simulink library "DTQC_lib"  (Simulink 7.5)
settings: Solver=ode45  StartTime=0.0  StopTime=10.0  RelTol=1e-3
values from neighbouring files (symbols this model uses):
  pDTQC_bool_AEBTrqSelect_C = Simulink.Parameter    [DTQC_par.m]
  pDTQC_Nm_ABSDelyOutTrq_C = Simulink.Parameter    [DTQC_par.m]
  pDTQC_Nm_AEBDelyOutTrq_C = Simulink.Parameter    [DTQC_par.m]
  pDTQC_Nm_AEBZeroTrq_C = Simulink.Parameter    [DTQC_par.m]
  pDTQC_Nm_ASRDelyOutTrq_C = Simulink.Parameter    [DTQC_par.m]
  pDTQC_Nm_MaxASRIntvTrq_C = Simulink.Parameter    [DTQC_par.m]
  pDTQC_Nm_MinASRIntvTrq_C = Simulink.Parameter    [DTQC_par.m]
  pDTQC_Nm_MSRDelyOutTrq_C = Simulink.Parameter    [DTQC_par.m]
  pDTQC_Nm_RBSDelyOutTrq_C = Simulink.Parameter    [DTQC_par.m]
  pDTQC_Nmps_ABSOutTrqLo_C = Simulink.Parameter    [DTQC_par.m]
  pDTQC_Nmps_ABSOutTrqUp_C = Simulink.Parameter    [DTQC_par.m]
  pDTQC_Nmps_AEBOutTrqLo_C = Simulink.Parameter    [DTQC_par.m]
  pDTQC_Nmps_AEBOutTrqUp_C = Simulink.Parameter    [DTQC_par.m]
  pDTQC_Nmps_ASROutTrqLo_C = Simulink.Parameter    [DTQC_par.m]
  pDTQC_Nmps_ASROutTrqUp_C = Simulink.Parameter    [DTQC_par.m]
  pDTQC_Nmps_MSROutTrqLo_C = Simulink.Parameter    [DTQC_par.m]
  pDTQC_Nmps_MSROutTrqUp_C = Simulink.Parameter    [DTQC_par.m]
  pDTQC_Nmps_RBSOutTrqLo_C = Simulink.Parameter    [DTQC_par.m]
  pDTQC_Nmps_RBSOutTrqUp_C = Simulink.Parameter    [DTQC_par.m]
libraries: BaseOperationLib_Browser x52, A0EV_Lib1 x9, simulink x1
settings Model: Creator=wuaibin  LastModifiedBy=wuaibin

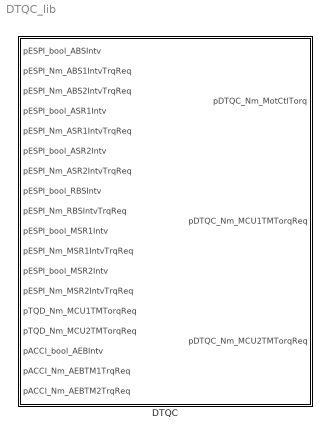
== system DTQC_lib ==
  DTQC : Subsystem  TreatAsAtomicUnit=on

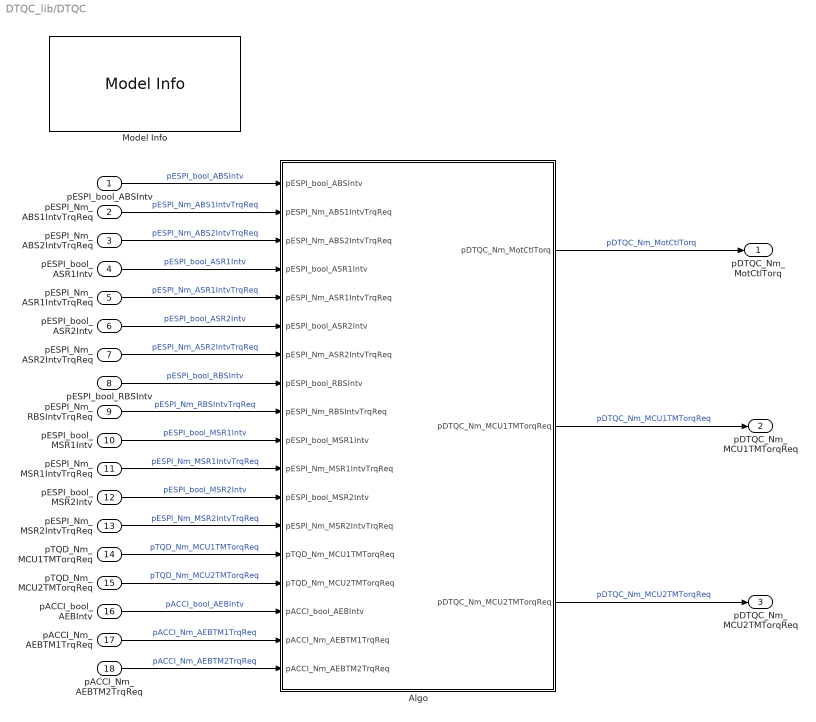
== system DTQC_lib/DTQC ==
  pESPI_bool_ABSIntv : Inport
  pESPI_Nm_ABS1IntvTrqReq : Inport  Port=2
  pESPI_Nm_ABS2IntvTrqReq : Inport  Port=3
  pESPI_bool_ASR1Intv : Inport  Port=4
  pESPI_Nm_ASR1IntvTrqReq : Inport  Port=5
  pESPI_bool_ASR2Intv : Inport  Port=6
  pESPI_Nm_ASR2IntvTrqReq : Inport  Port=7
  pESPI_bool_RBSIntv : Inport  Port=8
  pESPI_Nm_RBSIntvTrqReq : Inport  Port=9
  pESPI_bool_MSR1Intv : Inport  Port=10
  pESPI_Nm_MSR1IntvTrqReq : Inport  Port=11
  pESPI_bool_MSR2Intv : Inport  Port=12
  pESPI_Nm_MSR2IntvTrqReq : Inport  Port=13
  pTQD_Nm_MCU1TMTorqReq : Inport  Port=14
  pTQD_Nm_MCU2TMTorqReq : Inport  Port=15
  pACCI_bool_AEBIntv : Inport  Port=16
  pACCI_Nm_AEBTM1TrqReq : Inport  Port=17
  pACCI_Nm_AEBTM2TrqReq : Inport  Port=18
  Algo : Subsystem
  Model Info : simulink/Model-Wide Utilities/Model Info  SystemSampleTime=-1  InitialBlockCM=None  BlockCM=None  Frame=on  DisplayStringWithTags=Model Info\nCreated: %<Created>\nCreator: %<Creator>  HorizontalTextAlignment=Center  LeftAlignmentValue=0.5  SourceBlockDiagram=HQEV_HCU  TagMaxNumber=20
  pDTQC_Nm_MotCtlTorq : Outport  OutDataType=fixdt(1, 16)  OutScaling=2^0
  pDTQC_Nm_MCU1TMTorqReq : Outport  Port=2
  pDTQC_Nm_MCU2TMTorqReq : Outport  Port=3
  wires:
  pACCI_Nm_AEBTM2TrqReq/1 -> Algo/18(pACCI_Nm_AEBTM2TrqReq)  "pACCI_Nm_AEBTM2TrqReq"
  pACCI_Nm_AEBTM1TrqReq/1 -> Algo/17(pACCI_Nm_AEBTM1TrqReq)  "pACCI_Nm_AEBTM1TrqReq"
  pACCI_bool_AEBIntv/1 -> Algo/16(pACCI_bool_AEBIntv)  "pACCI_bool_AEBIntv"
  pTQD_Nm_MCU2TMTorqReq/1 -> Algo/15(pTQD_Nm_MCU2TMTorqReq)  "pTQD_Nm_MCU2TMTorqReq"
  pTQD_Nm_MCU1TMTorqReq/1 -> Algo/14(pTQD_Nm_MCU1TMTorqReq)  "pTQD_Nm_MCU1TMTorqReq"
  pESPI_Nm_MSR2IntvTrqReq/1 -> Algo/13(pESPI_Nm_MSR2IntvTrqReq)  "pESPI_Nm_MSR2IntvTrqReq"
  pESPI_bool_MSR2Intv/1 -> Algo/12(pESPI_bool_MSR2Intv)  "pESPI_bool_MSR2Intv"
  pESPI_Nm_MSR1IntvTrqReq/1 -> Algo/11(pESPI_Nm_MSR1IntvTrqReq)  "pESPI_Nm_MSR1IntvTrqReq"
  pESPI_bool_MSR1Intv/1 -> Algo/10(pESPI_bool_MSR1Intv)  "pESPI_bool_MSR1Intv"
  pESPI_Nm_RBSIntvTrqReq/1 -> Algo/9(pESPI_Nm_RBSIntvTrqReq)  "pESPI_Nm_RBSIntvTrqReq"
  pESPI_bool_RBSIntv/1 -> Algo/8(pESPI_bool_RBSIntv)  "pESPI_bool_RBSIntv"
  pESPI_Nm_ASR2IntvTrqReq/1 -> Algo/7(pESPI_Nm_ASR2IntvTrqReq)  "pESPI_Nm_ASR2IntvTrqReq"
  pESPI_bool_ASR2Intv/1 -> Algo/6(pESPI_bool_ASR2Intv)  "pESPI_bool_ASR2Intv"
  pESPI_Nm_ASR1IntvTrqReq/1 -> Algo/5(pESPI_Nm_ASR1IntvTrqReq)  "pESPI_Nm_ASR1IntvTrqReq"
  pESPI_bool_ASR1Intv/1 -> Algo/4(pESPI_bool_ASR1Intv)  "pESPI_bool_ASR1Intv"
  pESPI_Nm_ABS2IntvTrqReq/1 -> Algo/3(pESPI_Nm_ABS2IntvTrqReq)  "pESPI_Nm_ABS2IntvTrqReq"
  pESPI_Nm_ABS1IntvTrqReq/1 -> Algo/2(pESPI_Nm_ABS1IntvTrqReq)  "pESPI_Nm_ABS1IntvTrqReq"
  pESPI_bool_ABSIntv/1 -> Algo/1(pESPI_bool_ABSIntv)  "pESPI_bool_ABSIntv"
  Algo/3(pDTQC_Nm_MCU2TMTorqReq) -> pDTQC_Nm_MCU2TMTorqReq/1  "pDTQC_Nm_MCU2TMTorqReq"
  Algo/2(pDTQC_Nm_MCU1TMTorqReq) -> pDTQC_Nm_MCU1TMTorqReq/1  "pDTQC_Nm_MCU1TMTorqReq"
  Algo/1(pDTQC_Nm_MotCtlTorq) -> pDTQC_Nm_MotCtlTorq/1  "pDTQC_Nm_MotCtlTorq"

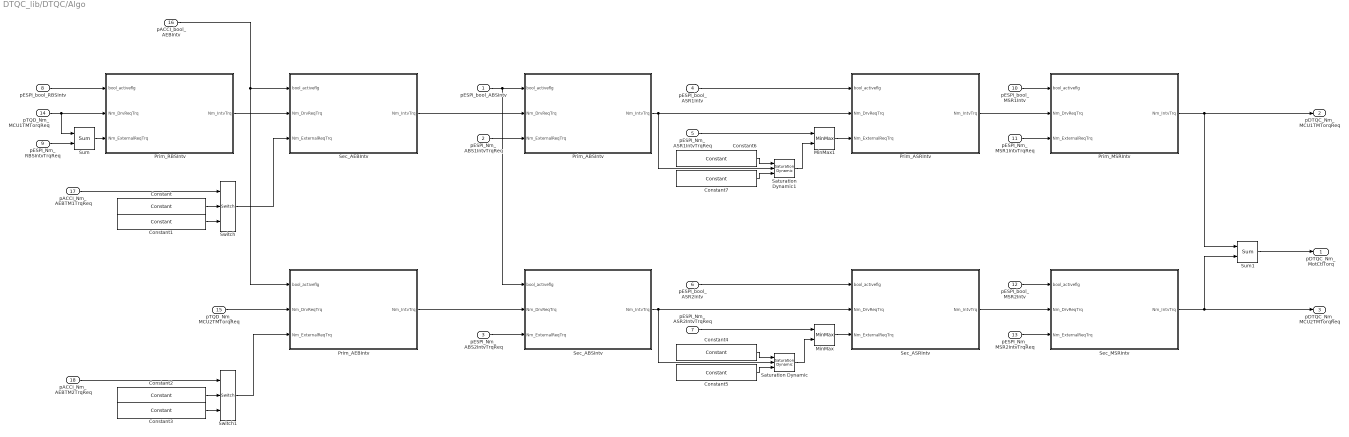
== system DTQC_lib/DTQC/Algo ==
  pESPI_bool_ABSIntv : Inport
  pESPI_Nm_ABS1IntvTrqReq : Inport  Port=2
  pESPI_Nm_ABS2IntvTrqReq : Inport  Port=3
  pESPI_bool_ASR1Intv : Inport  Port=4
  pESPI_Nm_ASR1IntvTrqReq : Inport  Port=5
  pESPI_bool_ASR2Intv : Inport  Port=6
  pESPI_Nm_ASR2IntvTrqReq : Inport  Port=7
  pESPI_bool_RBSIntv : Inport  Port=8
  pESPI_Nm_RBSIntvTrqReq : Inport  Port=9
  pESPI_bool_MSR1Intv : Inport  Port=10
  pESPI_Nm_MSR1IntvTrqReq : Inport  Port=11
  pESPI_bool_MSR2Intv : Inport  Port=12
  pESPI_Nm_MSR2IntvTrqReq : Inport  Port=13
  pTQD_Nm_MCU1TMTorqReq : Inport  Port=14
  pTQD_Nm_MCU2TMTorqReq : Inport  Port=15
  pACCI_bool_AEBIntv : Inport  Port=16
  pACCI_Nm_AEBTM1TrqReq : Inport  Port=17
  pACCI_Nm_AEBTM2TrqReq : Inport  Port=18
  Constant : BaseOperationLib_Browser/Sources&Sinks/Constant  Value=pDTQC_bool_AEBTrqSelect_C  OutMin=[]  OutMax=[]  OutDataType=fixdt(1, 16)  ConRadixGroup=Use specified scaling  OutScaling=2^0  OutDataTypeStr=Inherit: Inherit from 'Constant value'
  Constant1 : BaseOperationLib_Browser/Sources&Sinks/Constant  Value=pDTQC_Nm_AEBZeroTrq_C  OutMin=[]  OutMax=[]  OutDataType=fixdt(1, 16)  ConRadixGroup=Use specified scaling  OutScaling=2^0  OutDataTypeStr=Inherit: Inherit from 'Constant value'
  Constant2 : BaseOperationLib_Browser/Sources&Sinks/Constant  Value=pDTQC_bool_AEBTrqSelect_C  OutMin=[]  OutMax=[]  OutDataType=fixdt(1, 16)  ConRadixGroup=Use specified scaling  OutScaling=2^0  OutDataTypeStr=Inherit: Inherit from 'Constant value'
  Constant3 : BaseOperationLib_Browser/Sources&Sinks/Constant  Value=pDTQC_Nm_AEBZeroTrq_C  OutMin=[]  OutMax=[]  OutDataType=fixdt(1, 16)  ConRadixGroup=Use specified scaling  OutScaling=2^0  OutDataTypeStr=Inherit: Inherit from 'Constant value'
  Constant4 : BaseOperationLib_Browser/Sources&Sinks/Constant  Value=pDTQC_Nm_MaxASRIntvTrq_C  OutMin=[]  OutMax=[]  OutDataType=fixdt(1, 16)  ConRadixGroup=Use specified scaling  OutScaling=2^0  OutDataTypeStr=Inherit: Inherit from 'Constant value'
  Constant5 : BaseOperationLib_Browser/Sources&Sinks/Constant  Value=pDTQC_Nm_MinASRIntvTrq_C  OutMin=[]  OutMax=[]  OutDataType=fixdt(1, 16)  ConRadixGroup=Use specified scaling  OutScaling=2^0  OutDataTypeStr=Inherit: Inherit from 'Constant value'
  Constant6 : BaseOperationLib_Browser/Sources&Sinks/Constant  Value=pDTQC_Nm_MaxASRIntvTrq_C  OutMin=[]  OutMax=[]  OutDataType=fixdt(1, 16)  ConRadixGroup=Use specified scaling  OutScaling=2^0  OutDataTypeStr=Inherit: Inherit from 'Constant value'
  Constant7 : BaseOperationLib_Browser/Sources&Sinks/Constant  Value=pDTQC_Nm_MinASRIntvTrq_C  OutMin=[]  OutMax=[]  OutDataType=fixdt(1, 16)  ConRadixGroup=Use specified scaling  OutScaling=2^0  OutDataTypeStr=Inherit: Inherit from 'Constant value'
  MinMax : BaseOperationLib_Browser/Math Operations Changed/MinMax  Function=min  Inputs=2  InputSameDT=on  OutMin=[]  OutMax=[]  OutDataType=fixdt(1, 16)  OutScaling=2^0  SaturateOnIntegerOverflow=on
  MinMax1 : BaseOperationLib_Browser/Math Operations Changed/MinMax  Function=min  Inputs=2  InputSameDT=on  OutMin=[]  OutMax=[]  OutDataType=fixdt(1, 16)  OutScaling=2^0  SaturateOnIntegerOverflow=on
  Prim_ABSIntv : Subsystem
  Prim_AEBIntv : Subsystem
  Prim_ASRIntv : Subsystem
  Prim_MSRIntv : Subsystem
  Prim_RBSIntv : Subsystem
  Saturation Dynamic : BaseOperationLib_Browser/Discontinuities Unchanged/Saturation Dynamic  SystemSampleTime=-1  OutMin=[]  OutMax=[]  OutDataTypeStr=Inherit: Same as second input  OutDataType=fixdt(1, 16)  OutScaling=2^-10  DoSatur=on
  Saturation Dynamic1 : BaseOperationLib_Browser/Discontinuities Unchanged/Saturation Dynamic  SystemSampleTime=-1  OutMin=[]  OutMax=[]  OutDataTypeStr=Inherit: Same as second input  OutDataType=fixdt(1, 16)  OutScaling=2^-10  DoSatur=on
  Sec_ABSIntv : Subsystem
  Sec_AEBIntv : Subsystem
  Sec_ASRIntv : Subsystem
  Sec_MSRIntv : Subsystem
  Sum : BaseOperationLib_Browser/Math Operations Changed/Sum  Inputs=+-  InputSameDT=on  OutMin=[]  OutMax=[]  OutDataType=fixdt(1, 16)  OutScaling=2^0  SaturateOnIntegerOverflow=on
  Sum1 : BaseOperationLib_Browser/Math Operations Changed/Sum  Inputs=++  InputSameDT=on  OutMin=[]  OutMax=[]  OutDataType=fixdt(1, 16)  OutScaling=2^0  SaturateOnIntegerOverflow=on
  Switch : BaseOperationLib_Browser/Signal Routing Changed/Switch  Criteria=u2 ~= 0  Threshold=1  InputSameDT=on  OutMin=[]  OutMax=[]  OutDataType=fixdt(1,16,0)  OutScaling=[]  SaturateOnIntegerOverflow=on
  Switch1 : BaseOperationLib_Browser/Signal Routing Changed/Switch  Criteria=u2 ~= 0  Threshold=1  InputSameDT=on  OutMin=[]  OutMax=[]  OutDataType=fixdt(1,16,0)  OutScaling=[]  SaturateOnIntegerOverflow=on
  pDTQC_Nm_MotCtlTorq : Outport  OutDataType=fixdt(1, 16)  OutScaling=2^0
  pDTQC_Nm_MCU1TMTorqReq : Outport  Port=2
  pDTQC_Nm_MCU2TMTorqReq : Outport  Port=3
  wires:
  pESPI_Nm_ASR1IntvTrqReq/1 -> MinMax1/1
  Saturation Dynamic1/1 -> MinMax1/2
  Constant7/1 -> Saturation Dynamic1/3
  Constant6/1 -> Saturation Dynamic1/1
  MinMax1/1 -> Prim_ASRIntv/3(Nm_ExternalReqTrq)
  Constant5/1 -> Saturation Dynamic/3
  Constant4/1 -> Saturation Dynamic/1
  MinMax/1 -> Sec_ASRIntv/3(Nm_ExternalReqTrq)
  Saturation Dynamic/1 -> MinMax/2
  pESPI_Nm_ASR2IntvTrqReq/1 -> MinMax/1
  Sec_ASRIntv/1(Nm_IntvTrq) -> Sec_MSRIntv/2(Nm_DrvReqTrq)
  pESPI_bool_ASR2Intv/1 -> Sec_ASRIntv/1(bool_activeflg)
  pESPI_Nm_ABS2IntvTrqReq/1 -> Sec_ABSIntv/3(Nm_ExternalReqTrq)
  Prim_AEBIntv/1(Nm_IntvTrq) -> Sec_ABSIntv/2(Nm_DrvReqTrq)
  Sec_ABSIntv/1(Nm_IntvTrq) -> Saturation Dynamic/2, Sec_ASRIntv/2(Nm_DrvReqTrq)
  Prim_ASRIntv/1(Nm_IntvTrq) -> Prim_MSRIntv/2(Nm_DrvReqTrq)
  pESPI_bool_ASR1Intv/1 -> Prim_ASRIntv/1(bool_activeflg)
  Sec_AEBIntv/1(Nm_IntvTrq) -> Prim_ABSIntv/2(Nm_DrvReqTrq)
  Prim_ABSIntv/1(Nm_IntvTrq) -> Saturation Dynamic1/2, Prim_ASRIntv/2(Nm_DrvReqTrq)
  pESPI_Nm_ABS1IntvTrqReq/1 -> Prim_ABSIntv/3(Nm_ExternalReqTrq)
  pESPI_bool_ABSIntv/1 -> Sec_ABSIntv/1(bool_activeflg), Prim_ABSIntv/1(bool_activeflg)
  Sec_MSRIntv/1(Nm_IntvTrq) -> pDTQC_Nm_MCU2TMTorqReq/1, Sum1/2
  Prim_MSRIntv/1(Nm_IntvTrq) -> Sum1/1, pDTQC_Nm_MCU1TMTorqReq/1
  Switch1/1 -> Prim_AEBIntv/3(Nm_ExternalReqTrq)
  Switch/1 -> Sec_AEBIntv/3(Nm_ExternalReqTrq)
  pACCI_bool_AEBIntv/1 -> Prim_AEBIntv/1(bool_activeflg), Sec_AEBIntv/1(bool_activeflg)
  pTQD_Nm_MCU2TMTorqReq/1 -> Prim_AEBIntv/2(Nm_DrvReqTrq)
  Prim_RBSIntv/1(Nm_IntvTrq) -> Sec_AEBIntv/2(Nm_DrvReqTrq)
  Sum1/1 -> pDTQC_Nm_MotCtlTorq/1
  pESPI_Nm_MSR2IntvTrqReq/1 -> Sec_MSRIntv/3(Nm_ExternalReqTrq)
  pESPI_bool_MSR2Intv/1 -> Sec_MSRIntv/1(bool_activeflg)
  Constant3/1 -> Switch1/3
  pACCI_Nm_AEBTM2TrqReq/1 -> Switch1/1
  Constant2/1 -> Switch1/2
  Constant1/1 -> Switch/3
  pACCI_Nm_AEBTM1TrqReq/1 -> Switch/1
  Constant/1 -> Switch/2
  pESPI_Nm_RBSIntvTrqReq/1 -> Sum/2
  Sum/1 -> Prim_RBSIntv/3(Nm_ExternalReqTrq)
  pESPI_Nm_MSR1IntvTrqReq/1 -> Prim_MSRIntv/3(Nm_ExternalReqTrq)
  pESPI_bool_MSR1Intv/1 -> Prim_MSRIntv/1(bool_activeflg)
  pESPI_bool_RBSIntv/1 -> Prim_RBSIntv/1(bool_activeflg)
  pTQD_Nm_MCU1TMTorqReq/1 -> Sum/1, Prim_RBSIntv/2(Nm_DrvReqTrq)

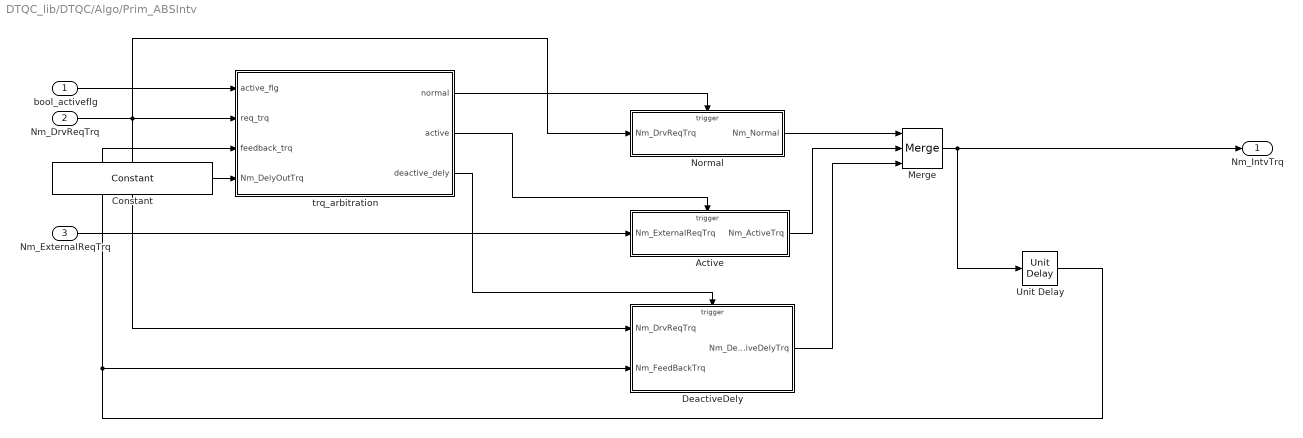
== system DTQC_lib/DTQC/Algo/Prim_ABSIntv ==
  bool_activeflg : Inport
  Nm_DrvReqTrq : Inport  Port=2
  Nm_ExternalReqTrq : Inport  Port=3
  Active : Subsystem
  Constant : BaseOperationLib_Browser/Sources&Sinks/Constant  Value=pDTQC_Nm_ABSDelyOutTrq_C  OutMin=[]  OutMax=[]  OutDataType=fixdt(1, 16)  ConRadixGroup=Use specified scaling  OutScaling=2^0  OutDataTypeStr=Inherit: Inherit from 'Constant value'
  DeactiveDely : Subsystem
  Merge : Merge  Inputs=3
  Normal : Subsystem
  Unit Delay : BaseOperationLib_Browser/Discrete Unchanged /Unit Delay  X0=0  SampleTime=-1
  trq_arbitration : Stateflow chart  TreatAsAtomicUnit=on
  Nm_IntvTrq : Outport  OutDataType=fixdt(1, 16)  OutScaling=2^0
  wires:
  bool_activeflg/1 -> trq_arbitration/1(active_flg)
  Nm_DrvReqTrq/1 -> trq_arbitration/2(req_trq), Normal/1(Nm_DrvReqTrq), DeactiveDely/1(Nm_DrvReqTrq)
  trq_arbitration/1(normal) -> Normal/Trigger
  trq_arbitration/2(active) -> Active/Trigger
  trq_arbitration/3(deactive_dely) -> DeactiveDely/Trigger
  Normal/1(Nm_Normal) -> Merge/1
  Active/1(Nm_ActiveTrq) -> Merge/2
  DeactiveDely/1(Nm_DeactiveDelyTrq) -> Merge/3
  Merge/1 -> Unit Delay/1, Nm_IntvTrq/1
  Unit Delay/1 -> trq_arbitration/3(feedback_trq), DeactiveDely/2(Nm_FeedBackTrq)
  Nm_ExternalReqTrq/1 -> Active/1(Nm_ExternalReqTrq)
  Constant/1 -> trq_arbitration/4(Nm_DelyOutTrq)

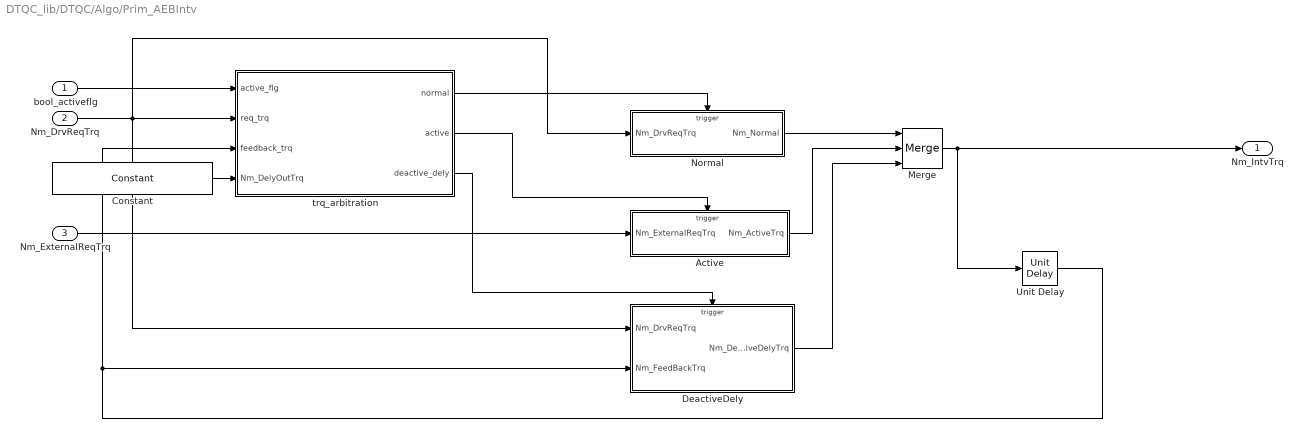
== system DTQC_lib/DTQC/Algo/Prim_AEBIntv ==
  bool_activeflg : Inport
  Nm_DrvReqTrq : Inport  Port=2
  Nm_ExternalReqTrq : Inport  Port=3
  Active : Subsystem
  Constant : BaseOperationLib_Browser/Sources&Sinks/Constant  Value=pDTQC_Nm_AEBDelyOutTrq_C  OutMin=[]  OutMax=[]  OutDataType=fixdt(1, 16)  ConRadixGroup=Use specified scaling  OutScaling=2^0  OutDataTypeStr=Inherit: Inherit from 'Constant value'
  DeactiveDely : Subsystem
  Merge : Merge  Inputs=3
  Normal : Subsystem
  Unit Delay : BaseOperationLib_Browser/Discrete Unchanged /Unit Delay  X0=0  SampleTime=-1
  trq_arbitration : Stateflow chart  TreatAsAtomicUnit=on
  Nm_IntvTrq : Outport  OutDataType=fixdt(1, 16)  OutScaling=2^0
  wires:
  Constant/1 -> trq_arbitration/4(Nm_DelyOutTrq)
  Nm_ExternalReqTrq/1 -> Active/1(Nm_ExternalReqTrq)
  Unit Delay/1 -> DeactiveDely/2(Nm_FeedBackTrq), trq_arbitration/3(feedback_trq)
  Merge/1 -> Nm_IntvTrq/1, Unit Delay/1
  DeactiveDely/1(Nm_DeactiveDelyTrq) -> Merge/3
  Active/1(Nm_ActiveTrq) -> Merge/2
  Normal/1(Nm_Normal) -> Merge/1
  trq_arbitration/3(deactive_dely) -> DeactiveDely/Trigger
  trq_arbitration/2(active) -> Active/Trigger
  trq_arbitration/1(normal) -> Normal/Trigger
  Nm_DrvReqTrq/1 -> DeactiveDely/1(Nm_DrvReqTrq), Normal/1(Nm_DrvReqTrq), trq_arbitration/2(req_trq)
  bool_activeflg/1 -> trq_arbitration/1(active_flg)

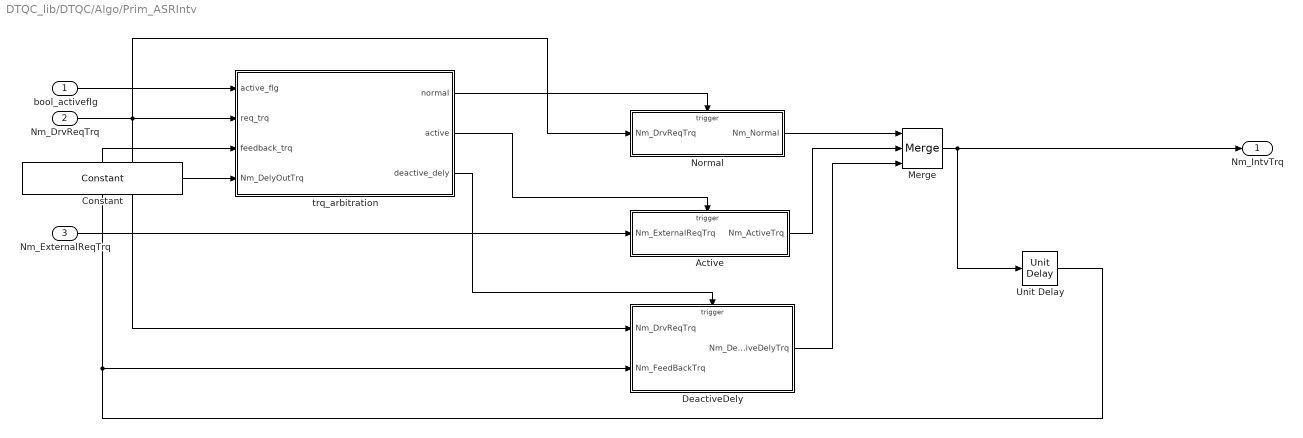
== system DTQC_lib/DTQC/Algo/Prim_ASRIntv ==
  bool_activeflg : Inport
  Nm_DrvReqTrq : Inport  Port=2
  Nm_ExternalReqTrq : Inport  Port=3
  Active : Subsystem
  Constant : BaseOperationLib_Browser/Sources&Sinks/Constant  Value=pDTQC_Nm_ASRDelyOutTrq_C  OutMin=[]  OutMax=[]  OutDataType=fixdt(1, 16)  ConRadixGroup=Use specified scaling  OutScaling=2^0  OutDataTypeStr=Inherit: Inherit from 'Constant value'
  DeactiveDely : Subsystem
  Merge : Merge  Inputs=3
  Normal : Subsystem
  Unit Delay : BaseOperationLib_Browser/Discrete Unchanged /Unit Delay  X0=0  SampleTime=-1
  trq_arbitration : Stateflow chart  TreatAsAtomicUnit=on
  Nm_IntvTrq : Outport  OutDataType=fixdt(1, 16)  OutScaling=2^0
  wires:
  Constant/1 -> trq_arbitration/4(Nm_DelyOutTrq)
  Nm_ExternalReqTrq/1 -> Active/1(Nm_ExternalReqTrq)
  Unit Delay/1 -> DeactiveDely/2(Nm_FeedBackTrq), trq_arbitration/3(feedback_trq)
  Merge/1 -> Nm_IntvTrq/1, Unit Delay/1
  DeactiveDely/1(Nm_DeactiveDelyTrq) -> Merge/3
  Active/1(Nm_ActiveTrq) -> Merge/2
  Normal/1(Nm_Normal) -> Merge/1
  trq_arbitration/3(deactive_dely) -> DeactiveDely/Trigger
  trq_arbitration/2(active) -> Active/Trigger
  trq_arbitration/1(normal) -> Normal/Trigger
  Nm_DrvReqTrq/1 -> DeactiveDely/1(Nm_DrvReqTrq), Normal/1(Nm_DrvReqTrq), trq_arbitration/2(req_trq)
  bool_activeflg/1 -> trq_arbitration/1(active_flg)

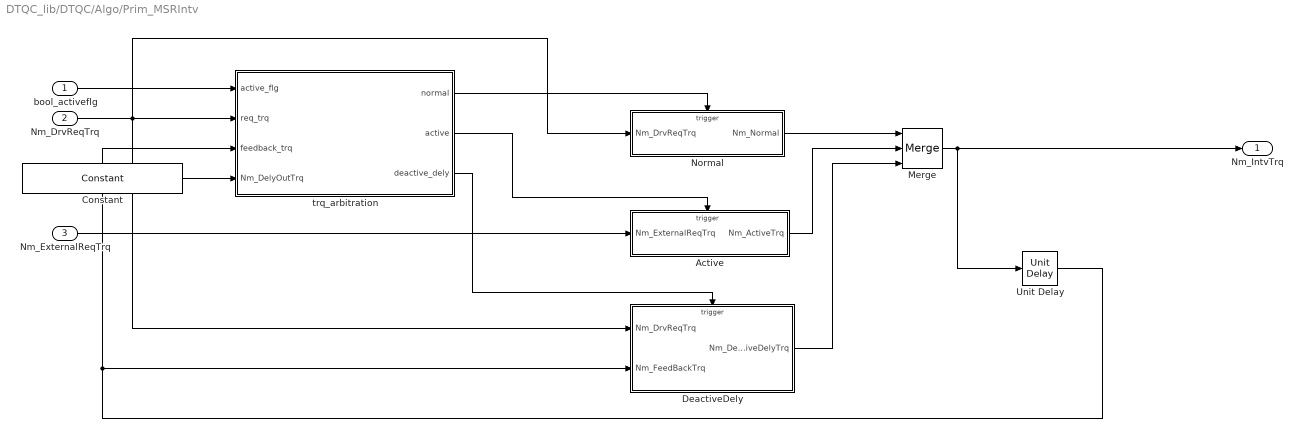
== system DTQC_lib/DTQC/Algo/Prim_MSRIntv ==
  bool_activeflg : Inport
  Nm_DrvReqTrq : Inport  Port=2
  Nm_ExternalReqTrq : Inport  Port=3
  Active : Subsystem
  Constant : BaseOperationLib_Browser/Sources&Sinks/Constant  Value=pDTQC_Nm_MSRDelyOutTrq_C  OutMin=[]  OutMax=[]  OutDataType=fixdt(1, 16)  ConRadixGroup=Use specified scaling  OutScaling=2^0  OutDataTypeStr=Inherit: Inherit from 'Constant value'
  DeactiveDely : Subsystem
  Merge : Merge  Inputs=3
  Normal : Subsystem
  Unit Delay : BaseOperationLib_Browser/Discrete Unchanged /Unit Delay  X0=0  SampleTime=-1
  trq_arbitration : Stateflow chart  TreatAsAtomicUnit=on
  Nm_IntvTrq : Outport  OutDataType=fixdt(1, 16)  OutScaling=2^0
  wires:
  bool_activeflg/1 -> trq_arbitration/1(active_flg)
  Nm_DrvReqTrq/1 -> trq_arbitration/2(req_trq), Normal/1(Nm_DrvReqTrq), DeactiveDely/1(Nm_DrvReqTrq)
  trq_arbitration/1(normal) -> Normal/Trigger
  trq_arbitration/2(active) -> Active/Trigger
  trq_arbitration/3(deactive_dely) -> DeactiveDely/Trigger
  Normal/1(Nm_Normal) -> Merge/1
  Active/1(Nm_ActiveTrq) -> Merge/2
  DeactiveDely/1(Nm_DeactiveDelyTrq) -> Merge/3
  Merge/1 -> Unit Delay/1, Nm_IntvTrq/1
  Unit Delay/1 -> trq_arbitration/3(feedback_trq), DeactiveDely/2(Nm_FeedBackTrq)
  Nm_ExternalReqTrq/1 -> Active/1(Nm_ExternalReqTrq)
  Constant/1 -> trq_arbitration/4(Nm_DelyOutTrq)

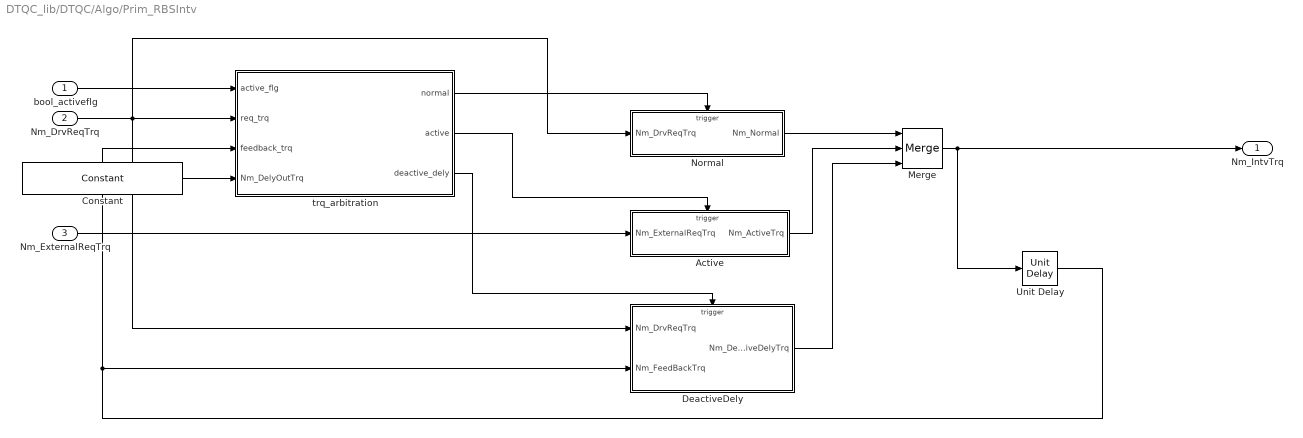
== system DTQC_lib/DTQC/Algo/Prim_RBSIntv ==
  bool_activeflg : Inport
  Nm_DrvReqTrq : Inport  Port=2
  Nm_ExternalReqTrq : Inport  Port=3
  Active : Subsystem
  Constant : BaseOperationLib_Browser/Sources&Sinks/Constant  Value=pDTQC_Nm_RBSDelyOutTrq_C  OutMin=[]  OutMax=[]  OutDataType=fixdt(1, 16)  ConRadixGroup=Use specified scaling  OutScaling=2^0  OutDataTypeStr=Inherit: Inherit from 'Constant value'
  DeactiveDely : Subsystem
  Merge : Merge  Inputs=3
  Normal : Subsystem
  Unit Delay : BaseOperationLib_Browser/Discrete Unchanged /Unit Delay  X0=0  SampleTime=-1
  trq_arbitration : Stateflow chart  TreatAsAtomicUnit=on
  Nm_IntvTrq : Outport  OutDataType=fixdt(1, 16)  OutScaling=2^0
  wires:
  Constant/1 -> trq_arbitration/4(Nm_DelyOutTrq)
  Nm_ExternalReqTrq/1 -> Active/1(Nm_ExternalReqTrq)
  Unit Delay/1 -> DeactiveDely/2(Nm_FeedBackTrq), trq_arbitration/3(feedback_trq)
  Merge/1 -> Nm_IntvTrq/1, Unit Delay/1
  DeactiveDely/1(Nm_DeactiveDelyTrq) -> Merge/3
  Active/1(Nm_ActiveTrq) -> Merge/2
  Normal/1(Nm_Normal) -> Merge/1
  trq_arbitration/3(deactive_dely) -> DeactiveDely/Trigger
  trq_arbitration/2(active) -> Active/Trigger
  trq_arbitration/1(normal) -> Normal/Trigger
  Nm_DrvReqTrq/1 -> DeactiveDely/1(Nm_DrvReqTrq), Normal/1(Nm_DrvReqTrq), trq_arbitration/2(req_trq)
  bool_activeflg/1 -> trq_arbitration/1(active_flg)

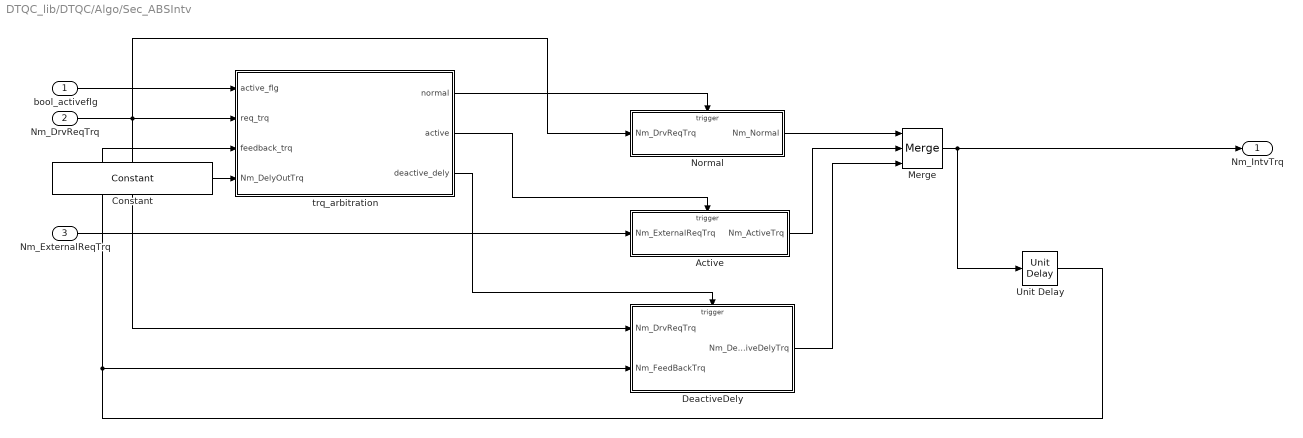
== system DTQC_lib/DTQC/Algo/Sec_ABSIntv ==
  bool_activeflg : Inport
  Nm_DrvReqTrq : Inport  Port=2
  Nm_ExternalReqTrq : Inport  Port=3
  Active : Subsystem
  Constant : BaseOperationLib_Browser/Sources&Sinks/Constant  Value=pDTQC_Nm_ABSDelyOutTrq_C  OutMin=[]  OutMax=[]  OutDataType=fixdt(1, 16)  ConRadixGroup=Use specified scaling  OutScaling=2^0  OutDataTypeStr=Inherit: Inherit from 'Constant value'
  DeactiveDely : Subsystem
  Merge : Merge  Inputs=3
  Normal : Subsystem
  Unit Delay : BaseOperationLib_Browser/Discrete Unchanged /Unit Delay  X0=0  SampleTime=-1
  trq_arbitration : Stateflow chart  TreatAsAtomicUnit=on
  Nm_IntvTrq : Outport  OutDataType=fixdt(1, 16)  OutScaling=2^0
  wires:
  Constant/1 -> trq_arbitration/4(Nm_DelyOutTrq)
  Nm_ExternalReqTrq/1 -> Active/1(Nm_ExternalReqTrq)
  Unit Delay/1 -> DeactiveDely/2(Nm_FeedBackTrq), trq_arbitration/3(feedback_trq)
  Merge/1 -> Nm_IntvTrq/1, Unit Delay/1
  DeactiveDely/1(Nm_DeactiveDelyTrq) -> Merge/3
  Active/1(Nm_ActiveTrq) -> Merge/2
  Normal/1(Nm_Normal) -> Merge/1
  trq_arbitration/3(deactive_dely) -> DeactiveDely/Trigger
  trq_arbitration/2(active) -> Active/Trigger
  trq_arbitration/1(normal) -> Normal/Trigger
  Nm_DrvReqTrq/1 -> DeactiveDely/1(Nm_DrvReqTrq), Normal/1(Nm_DrvReqTrq), trq_arbitration/2(req_trq)
  bool_activeflg/1 -> trq_arbitration/1(active_flg)

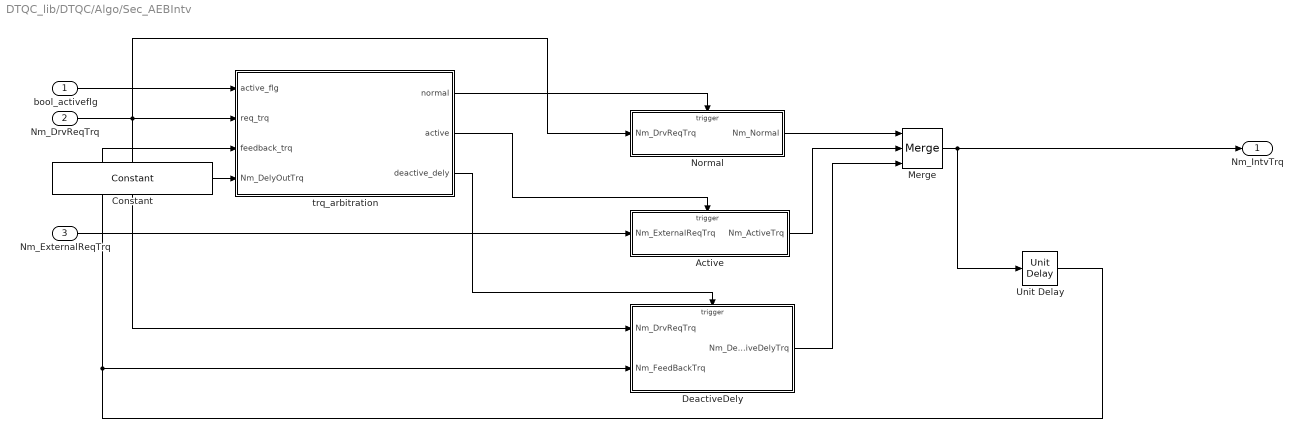
== system DTQC_lib/DTQC/Algo/Sec_AEBIntv ==
  bool_activeflg : Inport
  Nm_DrvReqTrq : Inport  Port=2
  Nm_ExternalReqTrq : Inport  Port=3
  Active : Subsystem
  Constant : BaseOperationLib_Browser/Sources&Sinks/Constant  Value=pDTQC_Nm_AEBDelyOutTrq_C  OutMin=[]  OutMax=[]  OutDataType=fixdt(1, 16)  ConRadixGroup=Use specified scaling  OutScaling=2^0  OutDataTypeStr=Inherit: Inherit from 'Constant value'
  DeactiveDely : Subsystem
  Merge : Merge  Inputs=3
  Normal : Subsystem
  Unit Delay : BaseOperationLib_Browser/Discrete Unchanged /Unit Delay  X0=0  SampleTime=-1
  trq_arbitration : Stateflow chart  TreatAsAtomicUnit=on
  Nm_IntvTrq : Outport  OutDataType=fixdt(1, 16)  OutScaling=2^0
  wires:
  bool_activeflg/1 -> trq_arbitration/1(active_flg)
  Nm_DrvReqTrq/1 -> trq_arbitration/2(req_trq), Normal/1(Nm_DrvReqTrq), DeactiveDely/1(Nm_DrvReqTrq)
  trq_arbitration/1(normal) -> Normal/Trigger
  trq_arbitration/2(active) -> Active/Trigger
  trq_arbitration/3(deactive_dely) -> DeactiveDely/Trigger
  Normal/1(Nm_Normal) -> Merge/1
  Active/1(Nm_ActiveTrq) -> Merge/2
  DeactiveDely/1(Nm_DeactiveDelyTrq) -> Merge/3
  Merge/1 -> Unit Delay/1, Nm_IntvTrq/1
  Unit Delay/1 -> trq_arbitration/3(feedback_trq), DeactiveDely/2(Nm_FeedBackTrq)
  Nm_ExternalReqTrq/1 -> Active/1(Nm_ExternalReqTrq)
  Constant/1 -> trq_arbitration/4(Nm_DelyOutTrq)

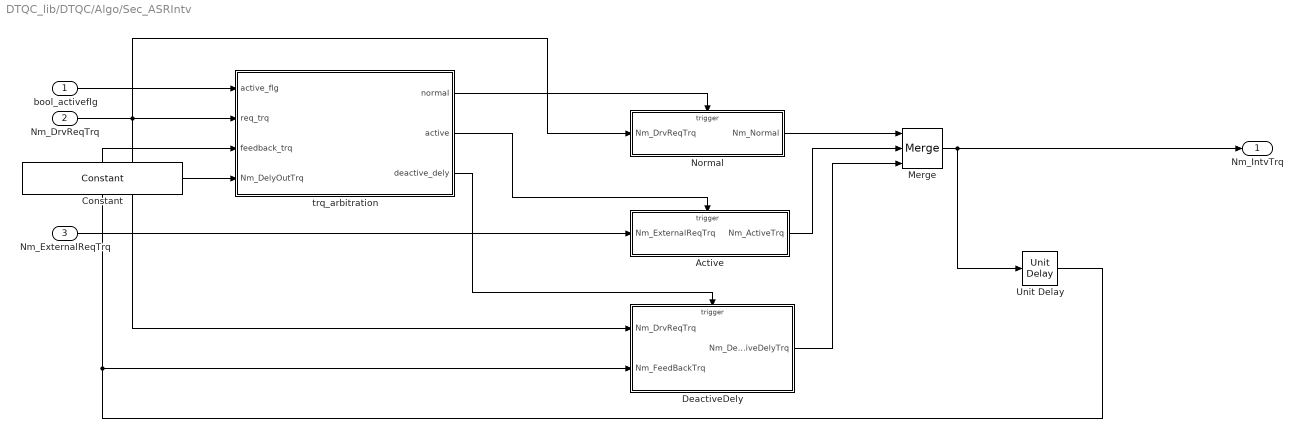
== system DTQC_lib/DTQC/Algo/Sec_ASRIntv ==
  bool_activeflg : Inport
  Nm_DrvReqTrq : Inport  Port=2
  Nm_ExternalReqTrq : Inport  Port=3
  Active : Subsystem
  Constant : BaseOperationLib_Browser/Sources&Sinks/Constant  Value=pDTQC_Nm_ASRDelyOutTrq_C  OutMin=[]  OutMax=[]  OutDataType=fixdt(1, 16)  ConRadixGroup=Use specified scaling  OutScaling=2^0  OutDataTypeStr=Inherit: Inherit from 'Constant value'
  DeactiveDely : Subsystem
  Merge : Merge  Inputs=3
  Normal : Subsystem
  Unit Delay : BaseOperationLib_Browser/Discrete Unchanged /Unit Delay  X0=0  SampleTime=-1
  trq_arbitration : Stateflow chart  TreatAsAtomicUnit=on
  Nm_IntvTrq : Outport  OutDataType=fixdt(1, 16)  OutScaling=2^0
  wires:
  bool_activeflg/1 -> trq_arbitration/1(active_flg)
  Nm_DrvReqTrq/1 -> trq_arbitration/2(req_trq), Normal/1(Nm_DrvReqTrq), DeactiveDely/1(Nm_DrvReqTrq)
  trq_arbitration/1(normal) -> Normal/Trigger
  trq_arbitration/2(active) -> Active/Trigger
  trq_arbitration/3(deactive_dely) -> DeactiveDely/Trigger
  Normal/1(Nm_Normal) -> Merge/1
  Active/1(Nm_ActiveTrq) -> Merge/2
  DeactiveDely/1(Nm_DeactiveDelyTrq) -> Merge/3
  Merge/1 -> Unit Delay/1, Nm_IntvTrq/1
  Unit Delay/1 -> trq_arbitration/3(feedback_trq), DeactiveDely/2(Nm_FeedBackTrq)
  Nm_ExternalReqTrq/1 -> Active/1(Nm_ExternalReqTrq)
  Constant/1 -> trq_arbitration/4(Nm_DelyOutTrq)

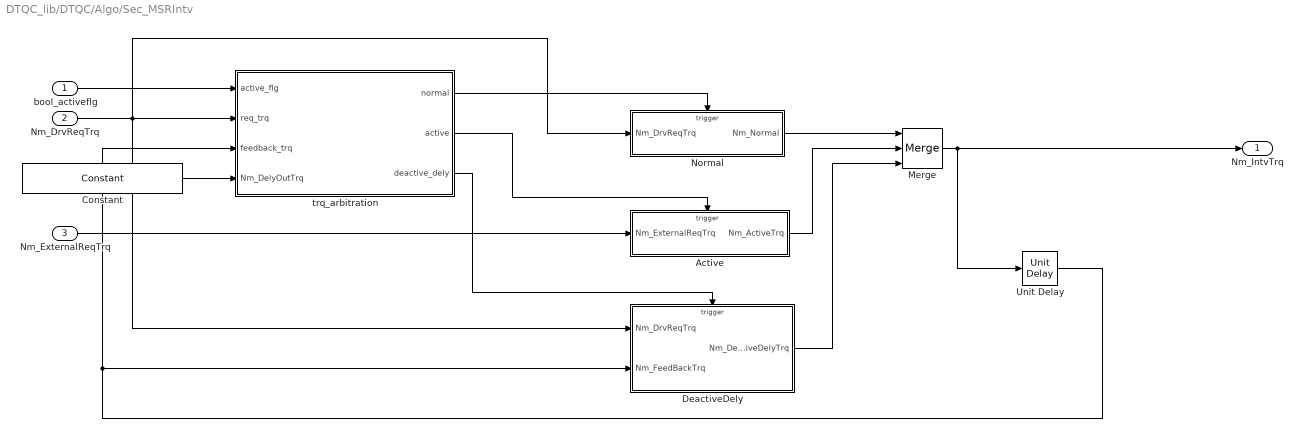
== system DTQC_lib/DTQC/Algo/Sec_MSRIntv ==
  bool_activeflg : Inport
  Nm_DrvReqTrq : Inport  Port=2
  Nm_ExternalReqTrq : Inport  Port=3
  Active : Subsystem
  Constant : BaseOperationLib_Browser/Sources&Sinks/Constant  Value=pDTQC_Nm_MSRDelyOutTrq_C  OutMin=[]  OutMax=[]  OutDataType=fixdt(1, 16)  ConRadixGroup=Use specified scaling  OutScaling=2^0  OutDataTypeStr=Inherit: Inherit from 'Constant value'
  DeactiveDely : Subsystem
  Merge : Merge  Inputs=3
  Normal : Subsystem
  Unit Delay : BaseOperationLib_Browser/Discrete Unchanged /Unit Delay  X0=0  SampleTime=-1
  trq_arbitration : Stateflow chart  TreatAsAtomicUnit=on
  Nm_IntvTrq : Outport  OutDataType=fixdt(1, 16)  OutScaling=2^0
  wires:
  Constant/1 -> trq_arbitration/4(Nm_DelyOutTrq)
  Nm_ExternalReqTrq/1 -> Active/1(Nm_ExternalReqTrq)
  Unit Delay/1 -> DeactiveDely/2(Nm_FeedBackTrq), trq_arbitration/3(feedback_trq)
  Merge/1 -> Nm_IntvTrq/1, Unit Delay/1
  DeactiveDely/1(Nm_DeactiveDelyTrq) -> Merge/3
  Active/1(Nm_ActiveTrq) -> Merge/2
  Normal/1(Nm_Normal) -> Merge/1
  trq_arbitration/3(deactive_dely) -> DeactiveDely/Trigger
  trq_arbitration/2(active) -> Active/Trigger
  trq_arbitration/1(normal) -> Normal/Trigger
  Nm_DrvReqTrq/1 -> DeactiveDely/1(Nm_DrvReqTrq), Normal/1(Nm_DrvReqTrq), trq_arbitration/2(req_trq)
  bool_activeflg/1 -> trq_arbitration/1(active_flg)

== system DTQC_lib/DTQC/Algo/Prim_ABSIntv/Active ==
  Nm_ExternalReqTrq : Inport  OutDataType=fixdt(1, 16)  OutScaling=2^0
  function : TriggerPort  TriggerType=function-call
  Nm_ActiveTrq : Outport  OutDataType=fixdt(1, 16)  OutScaling=2^0
  wires:
  Nm_ExternalReqTrq/1 -> Nm_ActiveTrq/1

== system DTQC_lib/DTQC/Algo/Prim_ABSIntv/DeactiveDely ==
  Nm_DrvReqTrq : Inport  OutDataType=fixdt(1, 16)  OutScaling=2^0
  Nm_FeedBackTrq : Inport  Port=2  OutDataType=fixdt(1, 16)  OutScaling=2^0
  function : TriggerPort  TriggerType=function-call
  Constant : BaseOperationLib_Browser/Sources&Sinks/Constant  Value=pDTQC_Nmps_ABSOutTrqUp_C  OutMin=[]  OutMax=[]  OutDataType=fixdt(1, 16)  ConRadixGroup=Use specified scaling  OutScaling=2^0  OutDataTypeStr=Inherit: Inherit from 'Constant value'
  Constant1 : BaseOperationLib_Browser/Sources&Sinks/Constant  Value=pDTQC_Nmps_ABSOutTrqLo_C  OutMin=[]  OutMax=[]  OutDataType=fixdt(1, 16)  ConRadixGroup=Use specified scaling  OutScaling=2^0  OutDataTypeStr=Inherit: Inherit from 'Constant value'
  RampLim : A0EV_Lib1/Filter & Ramp/RampLim  SystemSampleTime=-1
  Nm_DeactiveDelyTrq : Outport  OutDataType=fixdt(1, 16)  OutScaling=2^0
  wires:
  Nm_DrvReqTrq/1 -> RampLim/1
  Nm_FeedBackTrq/1 -> RampLim/2
  RampLim/1 -> Nm_DeactiveDelyTrq/1
  Constant/1 -> RampLim/3
  Constant1/1 -> RampLim/4

== system DTQC_lib/DTQC/Algo/Prim_ABSIntv/Normal ==
  Nm_DrvReqTrq : Inport  OutDataType=fixdt(1, 16)  OutScaling=2^0
  function : TriggerPort  TriggerType=function-call
  Nm_Normal : Outport  OutDataType=fixdt(1, 16)  OutScaling=2^0
  wires:
  Nm_DrvReqTrq/1 -> Nm_Normal/1

== system DTQC_lib/DTQC/Algo/Prim_AEBIntv/Active ==
  Nm_ExternalReqTrq : Inport  OutDataType=fixdt(1, 16)  OutScaling=2^0
  function : TriggerPort  TriggerType=function-call
  Nm_ActiveTrq : Outport  OutDataType=fixdt(1, 16)  OutScaling=2^0
  wires:
  Nm_ExternalReqTrq/1 -> Nm_ActiveTrq/1

== system DTQC_lib/DTQC/Algo/Prim_AEBIntv/DeactiveDely ==
  Nm_DrvReqTrq : Inport  OutDataType=fixdt(1, 16)  OutScaling=2^0
  Nm_FeedBackTrq : Inport  Port=2  OutDataType=fixdt(1, 16)  OutScaling=2^0
  function : TriggerPort  TriggerType=function-call
  Constant : BaseOperationLib_Browser/Sources&Sinks/Constant  Value=pDTQC_Nmps_AEBOutTrqUp_C  OutMin=[]  OutMax=[]  OutDataType=fixdt(1, 16)  ConRadixGroup=Use specified scaling  OutScaling=2^0  OutDataTypeStr=Inherit: Inherit from 'Constant value'
  Constant1 : BaseOperationLib_Browser/Sources&Sinks/Constant  Value=pDTQC_Nmps_AEBOutTrqLo_C  OutMin=[]  OutMax=[]  OutDataType=fixdt(1, 16)  ConRadixGroup=Use specified scaling  OutScaling=2^0  OutDataTypeStr=Inherit: Inherit from 'Constant value'
  RampLim : A0EV_Lib1/Filter & Ramp/RampLim  SystemSampleTime=-1
  Nm_DeactiveDelyTrq : Outport  OutDataType=fixdt(1, 16)  OutScaling=2^0
  wires:
  Constant1/1 -> RampLim/4
  Constant/1 -> RampLim/3
  RampLim/1 -> Nm_DeactiveDelyTrq/1
  Nm_FeedBackTrq/1 -> RampLim/2
  Nm_DrvReqTrq/1 -> RampLim/1

== system DTQC_lib/DTQC/Algo/Prim_AEBIntv/Normal ==
  Nm_DrvReqTrq : Inport  OutDataType=fixdt(1, 16)  OutScaling=2^0
  function : TriggerPort  TriggerType=function-call
  Nm_Normal : Outport  OutDataType=fixdt(1, 16)  OutScaling=2^0
  wires:
  Nm_DrvReqTrq/1 -> Nm_Normal/1

== system DTQC_lib/DTQC/Algo/Prim_ASRIntv/Active ==
  Nm_ExternalReqTrq : Inport  OutDataType=fixdt(1, 16)  OutScaling=2^0
  function : TriggerPort  TriggerType=function-call
  Nm_ActiveTrq : Outport  OutDataType=fixdt(1, 16)  OutScaling=2^0
  wires:
  Nm_ExternalReqTrq/1 -> Nm_ActiveTrq/1

== system DTQC_lib/DTQC/Algo/Prim_ASRIntv/DeactiveDely ==
  Nm_DrvReqTrq : Inport  OutDataType=fixdt(1, 16)  OutScaling=2^0
  Nm_FeedBackTrq : Inport  Port=2  OutDataType=fixdt(1, 16)  OutScaling=2^0
  function : TriggerPort  TriggerType=function-call
  Constant : BaseOperationLib_Browser/Sources&Sinks/Constant  Value=pDTQC_Nmps_ASROutTrqUp_C  OutMin=[]  OutMax=[]  OutDataType=fixdt(1, 16)  ConRadixGroup=Use specified scaling  OutScaling=2^0  OutDataTypeStr=Inherit: Inherit from 'Constant value'
  Constant1 : BaseOperationLib_Browser/Sources&Sinks/Constant  Value=pDTQC_Nmps_ASROutTrqLo_C  OutMin=[]  OutMax=[]  OutDataType=fixdt(1, 16)  ConRadixGroup=Use specified scaling  OutScaling=2^0  OutDataTypeStr=Inherit: Inherit from 'Constant value'
  RampLim : A0EV_Lib1/Filter & Ramp/RampLim  SystemSampleTime=-1
  Nm_DeactiveDelyTrq : Outport  OutDataType=fixdt(1, 16)  OutScaling=2^0
  wires:
  Constant1/1 -> RampLim/4
  Constant/1 -> RampLim/3
  RampLim/1 -> Nm_DeactiveDelyTrq/1
  Nm_FeedBackTrq/1 -> RampLim/2
  Nm_DrvReqTrq/1 -> RampLim/1

== system DTQC_lib/DTQC/Algo/Prim_ASRIntv/Normal ==
  Nm_DrvReqTrq : Inport  OutDataType=fixdt(1, 16)  OutScaling=2^0
  function : TriggerPort  TriggerType=function-call
  Nm_Normal : Outport  OutDataType=fixdt(1, 16)  OutScaling=2^0
  wires:
  Nm_DrvReqTrq/1 -> Nm_Normal/1

== system DTQC_lib/DTQC/Algo/Prim_MSRIntv/Active ==
  Nm_ExternalReqTrq : Inport  OutDataType=fixdt(1, 16)  OutScaling=2^0
  function : TriggerPort  TriggerType=function-call
  Nm_ActiveTrq : Outport  OutDataType=fixdt(1, 16)  OutScaling=2^0
  wires:
  Nm_ExternalReqTrq/1 -> Nm_ActiveTrq/1

== system DTQC_lib/DTQC/Algo/Prim_MSRIntv/DeactiveDely ==
  Nm_DrvReqTrq : Inport  OutDataType=fixdt(1, 16)  OutScaling=2^0
  Nm_FeedBackTrq : Inport  Port=2  OutDataType=fixdt(1, 16)  OutScaling=2^0
  function : TriggerPort  TriggerType=function-call
  Constant : BaseOperationLib_Browser/Sources&Sinks/Constant  Value=pDTQC_Nmps_MSROutTrqUp_C  OutMin=[]  OutMax=[]  OutDataType=fixdt(1, 16)  ConRadixGroup=Use specified scaling  OutScaling=2^0  OutDataTypeStr=Inherit: Inherit from 'Constant value'
  Constant1 : BaseOperationLib_Browser/Sources&Sinks/Constant  Value=pDTQC_Nmps_MSROutTrqLo_C  OutMin=[]  OutMax=[]  OutDataType=fixdt(1, 16)  ConRadixGroup=Use specified scaling  OutScaling=2^0  OutDataTypeStr=Inherit: Inherit from 'Constant value'
  RampLim : A0EV_Lib1/Filter & Ramp/RampLim  SystemSampleTime=-1
  Nm_DeactiveDelyTrq : Outport  OutDataType=fixdt(1, 16)  OutScaling=2^0
  wires:
  Nm_DrvReqTrq/1 -> RampLim/1
  Nm_FeedBackTrq/1 -> RampLim/2
  RampLim/1 -> Nm_DeactiveDelyTrq/1
  Constant/1 -> RampLim/3
  Constant1/1 -> RampLim/4

== system DTQC_lib/DTQC/Algo/Prim_MSRIntv/Normal ==
  Nm_DrvReqTrq : Inport  OutDataType=fixdt(1, 16)  OutScaling=2^0
  function : TriggerPort  TriggerType=function-call
  Nm_Normal : Outport  OutDataType=fixdt(1, 16)  OutScaling=2^0
  wires:
  Nm_DrvReqTrq/1 -> Nm_Normal/1

== system DTQC_lib/DTQC/Algo/Prim_RBSIntv/Active ==
  Nm_ExternalReqTrq : Inport  OutDataType=fixdt(1, 16)  OutScaling=2^0
  function : TriggerPort  TriggerType=function-call
  Nm_ActiveTrq : Outport  OutDataType=fixdt(1, 16)  OutScaling=2^0
  wires:
  Nm_ExternalReqTrq/1 -> Nm_ActiveTrq/1

== system DTQC_lib/DTQC/Algo/Prim_RBSIntv/DeactiveDely ==
  Nm_DrvReqTrq : Inport  OutDataType=fixdt(1, 16)  OutScaling=2^0
  Nm_FeedBackTrq : Inport  Port=2  OutDataType=fixdt(1, 16)  OutScaling=2^0
  function : TriggerPort  TriggerType=function-call
  Constant : BaseOperationLib_Browser/Sources&Sinks/Constant  Value=pDTQC_Nmps_RBSOutTrqUp_C  OutMin=[]  OutMax=[]  OutDataType=fixdt(1, 16)  ConRadixGroup=Use specified scaling  OutScaling=2^0  OutDataTypeStr=Inherit: Inherit from 'Constant value'
  Constant1 : BaseOperationLib_Browser/Sources&Sinks/Constant  Value=pDTQC_Nmps_RBSOutTrqLo_C  OutMin=[]  OutMax=[]  OutDataType=fixdt(1, 16)  ConRadixGroup=Use specified scaling  OutScaling=2^0  OutDataTypeStr=Inherit: Inherit from 'Constant value'
  RampLim : A0EV_Lib1/Filter & Ramp/RampLim  SystemSampleTime=-1
  Nm_DeactiveDelyTrq : Outport  OutDataType=fixdt(1, 16)  OutScaling=2^0
  wires:
  Constant1/1 -> RampLim/4
  Constant/1 -> RampLim/3
  RampLim/1 -> Nm_DeactiveDelyTrq/1
  Nm_FeedBackTrq/1 -> RampLim/2
  Nm_DrvReqTrq/1 -> RampLim/1

== system DTQC_lib/DTQC/Algo/Prim_RBSIntv/Normal ==
  Nm_DrvReqTrq : Inport  OutDataType=fixdt(1, 16)  OutScaling=2^0
  function : TriggerPort  TriggerType=function-call
  Nm_Normal : Outport  OutDataType=fixdt(1, 16)  OutScaling=2^0
  wires:
  Nm_DrvReqTrq/1 -> Nm_Normal/1

== system DTQC_lib/DTQC/Algo/Sec_ABSIntv/Active ==
  Nm_ExternalReqTrq : Inport  OutDataType=fixdt(1, 16)  OutScaling=2^0
  function : TriggerPort  TriggerType=function-call
  Nm_ActiveTrq : Outport  OutDataType=fixdt(1, 16)  OutScaling=2^0
  wires:
  Nm_ExternalReqTrq/1 -> Nm_ActiveTrq/1

== system DTQC_lib/DTQC/Algo/Sec_ABSIntv/DeactiveDely ==
  Nm_DrvReqTrq : Inport  OutDataType=fixdt(1, 16)  OutScaling=2^0
  Nm_FeedBackTrq : Inport  Port=2  OutDataType=fixdt(1, 16)  OutScaling=2^0
  function : TriggerPort  TriggerType=function-call
  Constant : BaseOperationLib_Browser/Sources&Sinks/Constant  Value=pDTQC_Nmps_ABSOutTrqUp_C  OutMin=[]  OutMax=[]  OutDataType=fixdt(1, 16)  ConRadixGroup=Use specified scaling  OutScaling=2^0  OutDataTypeStr=Inherit: Inherit from 'Constant value'
  Constant1 : BaseOperationLib_Browser/Sources&Sinks/Constant  Value=pDTQC_Nmps_ABSOutTrqLo_C  OutMin=[]  OutMax=[]  OutDataType=fixdt(1, 16)  ConRadixGroup=Use specified scaling  OutScaling=2^0  OutDataTypeStr=Inherit: Inherit from 'Constant value'
  RampLim : A0EV_Lib1/Filter & Ramp/RampLim  SystemSampleTime=-1
  Nm_DeactiveDelyTrq : Outport  OutDataType=fixdt(1, 16)  OutScaling=2^0
  wires:
  Constant1/1 -> RampLim/4
  Constant/1 -> RampLim/3
  RampLim/1 -> Nm_DeactiveDelyTrq/1
  Nm_FeedBackTrq/1 -> RampLim/2
  Nm_DrvReqTrq/1 -> RampLim/1

== system DTQC_lib/DTQC/Algo/Sec_ABSIntv/Normal ==
  Nm_DrvReqTrq : Inport  OutDataType=fixdt(1, 16)  OutScaling=2^0
  function : TriggerPort  TriggerType=function-call
  Nm_Normal : Outport  OutDataType=fixdt(1, 16)  OutScaling=2^0
  wires:
  Nm_DrvReqTrq/1 -> Nm_Normal/1

== system DTQC_lib/DTQC/Algo/Sec_AEBIntv/Active ==
  Nm_ExternalReqTrq : Inport  OutDataType=fixdt(1, 16)  OutScaling=2^0
  function : TriggerPort  TriggerType=function-call
  Nm_ActiveTrq : Outport  OutDataType=fixdt(1, 16)  OutScaling=2^0
  wires:
  Nm_ExternalReqTrq/1 -> Nm_ActiveTrq/1

== system DTQC_lib/DTQC/Algo/Sec_AEBIntv/DeactiveDely ==
  Nm_DrvReqTrq : Inport  OutDataType=fixdt(1, 16)  OutScaling=2^0
  Nm_FeedBackTrq : Inport  Port=2  OutDataType=fixdt(1, 16)  OutScaling=2^0
  function : TriggerPort  TriggerType=function-call
  Constant : BaseOperationLib_Browser/Sources&Sinks/Constant  Value=pDTQC_Nmps_AEBOutTrqUp_C  OutMin=[]  OutMax=[]  OutDataType=fixdt(1, 16)  ConRadixGroup=Use specified scaling  OutScaling=2^0  OutDataTypeStr=Inherit: Inherit from 'Constant value'
  Constant1 : BaseOperationLib_Browser/Sources&Sinks/Constant  Value=pDTQC_Nmps_AEBOutTrqLo_C  OutMin=[]  OutMax=[]  OutDataType=fixdt(1, 16)  ConRadixGroup=Use specified scaling  OutScaling=2^0  OutDataTypeStr=Inherit: Inherit from 'Constant value'
  RampLim : A0EV_Lib1/Filter & Ramp/RampLim  SystemSampleTime=-1
  Nm_DeactiveDelyTrq : Outport  OutDataType=fixdt(1, 16)  OutScaling=2^0
  wires:
  Nm_DrvReqTrq/1 -> RampLim/1
  Nm_FeedBackTrq/1 -> RampLim/2
  RampLim/1 -> Nm_DeactiveDelyTrq/1
  Constant/1 -> RampLim/3
  Constant1/1 -> RampLim/4

== system DTQC_lib/DTQC/Algo/Sec_AEBIntv/Normal ==
  Nm_DrvReqTrq : Inport  OutDataType=fixdt(1, 16)  OutScaling=2^0
  function : TriggerPort  TriggerType=function-call
  Nm_Normal : Outport  OutDataType=fixdt(1, 16)  OutScaling=2^0
  wires:
  Nm_DrvReqTrq/1 -> Nm_Normal/1

== system DTQC_lib/DTQC/Algo/Sec_ASRIntv/Active ==
  Nm_ExternalReqTrq : Inport  OutDataType=fixdt(1, 16)  OutScaling=2^0
  function : TriggerPort  TriggerType=function-call
  Nm_ActiveTrq : Outport  OutDataType=fixdt(1, 16)  OutScaling=2^0
  wires:
  Nm_ExternalReqTrq/1 -> Nm_ActiveTrq/1

== system DTQC_lib/DTQC/Algo/Sec_ASRIntv/DeactiveDely ==
  Nm_DrvReqTrq : Inport  OutDataType=fixdt(1, 16)  OutScaling=2^0
  Nm_FeedBackTrq : Inport  Port=2  OutDataType=fixdt(1, 16)  OutScaling=2^0
  function : TriggerPort  TriggerType=function-call
  Constant : BaseOperationLib_Browser/Sources&Sinks/Constant  Value=pDTQC_Nmps_ASROutTrqUp_C  OutMin=[]  OutMax=[]  OutDataType=fixdt(1, 16)  ConRadixGroup=Use specified scaling  OutScaling=2^0  OutDataTypeStr=Inherit: Inherit from 'Constant value'
  Constant1 : BaseOperationLib_Browser/Sources&Sinks/Constant  Value=pDTQC_Nmps_ASROutTrqLo_C  OutMin=[]  OutMax=[]  OutDataType=fixdt(1, 16)  ConRadixGroup=Use specified scaling  OutScaling=2^0  OutDataTypeStr=Inherit: Inherit from 'Constant value'
  RampLim : A0EV_Lib1/Filter & Ramp/RampLim  SystemSampleTime=-1
  Nm_DeactiveDelyTrq : Outport  OutDataType=fixdt(1, 16)  OutScaling=2^0
  wires:
  Nm_DrvReqTrq/1 -> RampLim/1
  Nm_FeedBackTrq/1 -> RampLim/2
  RampLim/1 -> Nm_DeactiveDelyTrq/1
  Constant/1 -> RampLim/3
  Constant1/1 -> RampLim/4

== system DTQC_lib/DTQC/Algo/Sec_ASRIntv/Normal ==
  Nm_DrvReqTrq : Inport  OutDataType=fixdt(1, 16)  OutScaling=2^0
  function : TriggerPort  TriggerType=function-call
  Nm_Normal : Outport  OutDataType=fixdt(1, 16)  OutScaling=2^0
  wires:
  Nm_DrvReqTrq/1 -> Nm_Normal/1

== system DTQC_lib/DTQC/Algo/Sec_MSRIntv/Active ==
  Nm_ExternalReqTrq : Inport  OutDataType=fixdt(1, 16)  OutScaling=2^0
  function : TriggerPort  TriggerType=function-call
  Nm_ActiveTrq : Outport  OutDataType=fixdt(1, 16)  OutScaling=2^0
  wires:
  Nm_ExternalReqTrq/1 -> Nm_ActiveTrq/1

== system DTQC_lib/DTQC/Algo/Sec_MSRIntv/DeactiveDely ==
  Nm_DrvReqTrq : Inport  OutDataType=fixdt(1, 16)  OutScaling=2^0
  Nm_FeedBackTrq : Inport  Port=2  OutDataType=fixdt(1, 16)  OutScaling=2^0
  function : TriggerPort  TriggerType=function-call
  Constant : BaseOperationLib_Browser/Sources&Sinks/Constant  Value=pDTQC_Nmps_MSROutTrqUp_C  OutMin=[]  OutMax=[]  OutDataType=fixdt(1, 16)  ConRadixGroup=Use specified scaling  OutScaling=2^0  OutDataTypeStr=Inherit: Inherit from 'Constant value'
  Constant1 : BaseOperationLib_Browser/Sources&Sinks/Constant  Value=pDTQC_Nmps_MSROutTrqLo_C  OutMin=[]  OutMax=[]  OutDataType=fixdt(1, 16)  ConRadixGroup=Use specified scaling  OutScaling=2^0  OutDataTypeStr=Inherit: Inherit from 'Constant value'
  RampLim : A0EV_Lib1/Filter & Ramp/RampLim  SystemSampleTime=-1
  Nm_DeactiveDelyTrq : Outport  OutDataType=fixdt(1, 16)  OutScaling=2^0
  wires:
  Constant1/1 -> RampLim/4
  Constant/1 -> RampLim/3
  RampLim/1 -> Nm_DeactiveDelyTrq/1
  Nm_FeedBackTrq/1 -> RampLim/2
  Nm_DrvReqTrq/1 -> RampLim/1

== system DTQC_lib/DTQC/Algo/Sec_MSRIntv/Normal ==
  Nm_DrvReqTrq : Inport  OutDataType=fixdt(1, 16)  OutScaling=2^0
  function : TriggerPort  TriggerType=function-call
  Nm_Normal : Outport  OutDataType=fixdt(1, 16)  OutScaling=2^0
  wires:
  Nm_DrvReqTrq/1 -> Nm_Normal/1

== stateflow chart DTQC/Algo/Prim_ABSIntv/trq_arbitration ==
  state normal
    en:normal;
    du:normal;
  state active
    en:active;
    du:active;
  state deactive_dely
    en:deactive_dely;
    du:deactive_dely;
  (default) -> normal
  normal -> active : [active_flg==true]
  active -> deactive_dely : [active_flg==false]
  deactive_dely -> normal [order 1] : [abs(req_trq-feedback_trq)<=Nm_DelyOutTrq]
  deactive_dely -> active [order 2] : [active_flg==true]
  data: active_flg input double; req_trq input double; feedback_trq input double; Nm_DelyOutTrq input double
  events: normal output FUNCTION_CALL_EVENT; active output FUNCTION_CALL_EVENT; deactive_dely output FUNCTION_CALL_EVENT

== stateflow chart DTQC/Algo/Prim_ASRIntv/trq_arbitration ==
  state normal
    en:normal;
    du:normal;
  state active
    en:active;
    du:active;
  state deactive_dely
    en:deactive_dely;
    du:deactive_dely;
  (default) -> normal
  normal -> active : [active_flg==true]
  active -> deactive_dely : [active_flg==false]
  deactive_dely -> normal [order 1] : [abs(req_trq-feedback_trq)<=Nm_DelyOutTrq]
  deactive_dely -> active [order 2] : [active_flg==true]
  data: active_flg input double; req_trq input double; feedback_trq input double; Nm_DelyOutTrq input double
  events: normal output FUNCTION_CALL_EVENT; active output FUNCTION_CALL_EVENT; deactive_dely output FUNCTION_CALL_EVENT

== stateflow chart DTQC/Algo/Prim_MSRIntv/trq_arbitration ==
  state normal
    en:normal;
    du:normal;
  state active
    en:active;
    du:active;
  state deactive_dely
    en:deactive_dely;
    du:deactive_dely;
  (default) -> normal
  normal -> active : [active_flg==true]
  active -> deactive_dely : [active_flg==false]
  deactive_dely -> normal [order 1] : [abs(req_trq-feedback_trq)<=Nm_DelyOutTrq]
  deactive_dely -> active [order 2] : [active_flg==true]
  data: active_flg input double; req_trq input double; feedback_trq input double; Nm_DelyOutTrq input double
  events: normal output FUNCTION_CALL_EVENT; active output FUNCTION_CALL_EVENT; deactive_dely output FUNCTION_CALL_EVENT

== stateflow chart DTQC/Algo/Prim_RBSIntv/trq_arbitration ==
  state normal
    en:normal;
    du:normal;
  state active
    en:active;
    du:active;
  state deactive_dely
    en:deactive_dely;
    du:deactive_dely;
  (default) -> normal
  normal -> active : [active_flg==true]
  active -> deactive_dely : [active_flg==false]
  deactive_dely -> normal [order 1] : [abs(req_trq-feedback_trq)<=Nm_DelyOutTrq]
  deactive_dely -> active [order 2] : [active_flg==true]
  data: active_flg input double; req_trq input double; feedback_trq input double; Nm_DelyOutTrq input double
  events: normal output FUNCTION_CALL_EVENT; active output FUNCTION_CALL_EVENT; deactive_dely output FUNCTION_CALL_EVENT

== stateflow chart DTQC/Algo/Prim_AEBIntv/trq_arbitration ==
  state normal
    en:normal;
    du:normal;
  state active
    en:active;
    du:active;
  state deactive_dely
    en:deactive_dely;
    du:deactive_dely;
  (default) -> normal
  normal -> active : [active_flg==true]
  active -> deactive_dely : [active_flg==false]
  deactive_dely -> normal [order 1] : [abs(req_trq-feedback_trq)<=Nm_DelyOutTrq]
  deactive_dely -> active [order 2] : [active_flg==true]
  data: active_flg input double; req_trq input double; feedback_trq input double; Nm_DelyOutTrq input double
  events: normal output FUNCTION_CALL_EVENT; active output FUNCTION_CALL_EVENT; deactive_dely output FUNCTION_CALL_EVENT

== stateflow chart DTQC/Algo/Sec_ASRIntv/trq_arbitration ==
  state normal
    en:normal;
    du:normal;
  state active
    en:active;
    du:active;
  state deactive_dely
    en:deactive_dely;
    du:deactive_dely;
  (default) -> normal
  normal -> active : [active_flg==true]
  active -> deactive_dely : [active_flg==false]
  deactive_dely -> normal [order 1] : [abs(req_trq-feedback_trq)<=Nm_DelyOutTrq]
  deactive_dely -> active [order 2] : [active_flg==true]
  data: active_flg input double; req_trq input double; feedback_trq input double; Nm_DelyOutTrq input double
  events: normal output FUNCTION_CALL_EVENT; active output FUNCTION_CALL_EVENT; deactive_dely output FUNCTION_CALL_EVENT

== stateflow chart DTQC/Algo/Sec_MSRIntv/trq_arbitration ==
  state normal
    en:normal;
    du:normal;
  state active
    en:active;
    du:active;
  state deactive_dely
    en:deactive_dely;
    du:deactive_dely;
  (default) -> normal
  normal -> active : [active_flg==true]
  active -> deactive_dely : [active_flg==false]
  deactive_dely -> normal [order 1] : [abs(req_trq-feedback_trq)<=Nm_DelyOutTrq]
  deactive_dely -> active [order 2] : [active_flg==true]
  data: active_flg input double; req_trq input double; feedback_trq input double; Nm_DelyOutTrq input double
  events: normal output FUNCTION_CALL_EVENT; active output FUNCTION_CALL_EVENT; deactive_dely output FUNCTION_CALL_EVENT

== stateflow chart DTQC/Algo/Sec_ABSIntv/trq_arbitration ==
  state normal
    en:normal;
    du:normal;
  state active
    en:active;
    du:active;
  state deactive_dely
    en:deactive_dely;
    du:deactive_dely;
  (default) -> normal
  normal -> active : [active_flg==true]
  active -> deactive_dely : [active_flg==false]
  deactive_dely -> normal [order 1] : [abs(req_trq-feedback_trq)<=Nm_DelyOutTrq]
  deactive_dely -> active [order 2] : [active_flg==true]
  data: active_flg input double; req_trq input double; feedback_trq input double; Nm_DelyOutTrq input double
  events: normal output FUNCTION_CALL_EVENT; active output FUNCTION_CALL_EVENT; deactive_dely output FUNCTION_CALL_EVENT

== stateflow chart DTQC/Algo/Sec_AEBIntv/trq_arbitration ==
  state normal
    en:normal;
    du:normal;
  state active
    en:active;
    du:active;
  state deactive_dely
    en:deactive_dely;
    du:deactive_dely;
  (default) -> normal
  normal -> active : [active_flg==true]
  active -> deactive_dely : [active_flg==false]
  deactive_dely -> normal [order 1] : [abs(req_trq-feedback_trq)<=Nm_DelyOutTrq]
  deactive_dely -> active [order 2] : [active_flg==true]
  data: active_flg input double; req_trq input double; feedback_trq input double; Nm_DelyOutTrq input double
  events: normal output FUNCTION_CALL_EVENT; active output FUNCTION_CALL_EVENT; deactive_dely output FUNCTION_CALL_EVENT
